simulink library "groundStation001_cl"  (R2018b)
settings: Solver=VariableStepAuto  StartTime=0.0  StopTime=10.0  RelTol=1e-3
values from neighbouring files (symbols this model uses):
  env = ENV.env    [groundStation001_ts.m]    (also in groundStation001_ts2.m; groundStation001_ts3.m)
  gndStn = OCT.sixDoFStation    [groundStation001_ts3.m]
libraries: thrAttachPtKinematics_ul x3, tethersMoment_cl x2, vrlib x1, eulAng2RotMat_ul x1, circulationForce_ul x1, sixDoFDynamics_ul x1, tether000_cl x1, variableBuoyancy_ul x1, winch_cl x1
settings Model: Creator=Erin B  LastModifiedBy=mcobb

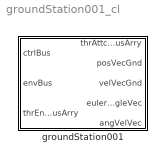
== system groundStation001_cl ==
  groundStation001 : Subsystem  mask{gs=gndStn, e=0, numNodes=0}
      mask prompts: gs "Ground Station"; e "Environmetnt"; numNodes "Number of anchor tether nodes"
      mask init:
      | groundStation001_init

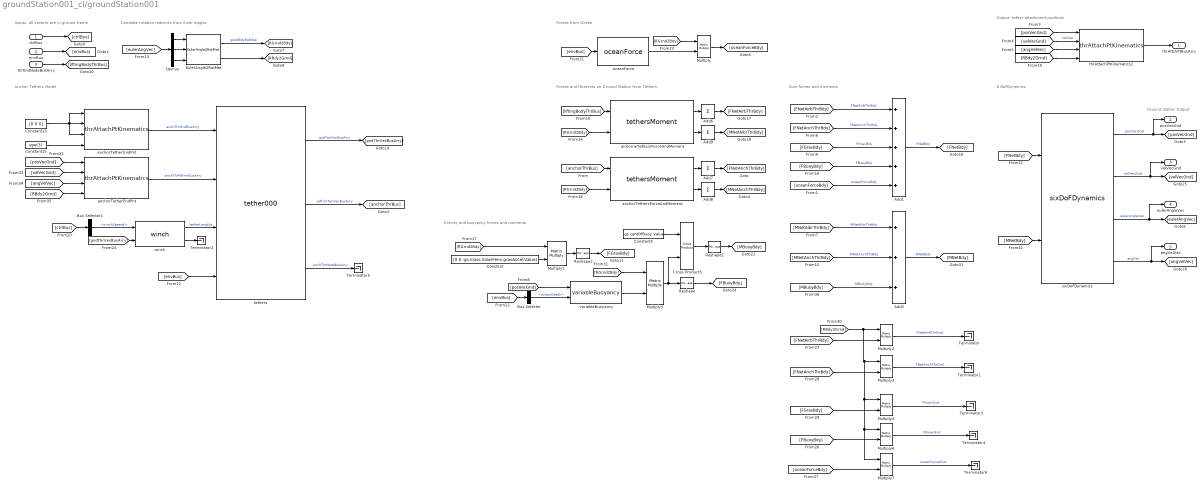
== system groundStation001_cl/groundStation001 ==
  note: Ground Station Output
  note: Anchor Tethers Model
  note: Forces and Moments on Ground Station from Tethers
  note: Output: tether attachment positions
  note: Inputs, all vectors are in ground frame
  note: Calculate rotation matrices from Euler angles
  note: Sum forces and moments
  note: Gravity and buoyancy forces and moments
  note: 6 DoFDynamics
  note: Forces from Ocean
  ctrlBus : Inport  OutDataTypeStr=Bus: gndStnCtrlBus
  envBus : Inport  Port=2  OutDataTypeStr=Bus: envBus
  thrEndNodeBusArry : Inport  Port=3
  Add1 : Sum  Inputs=+++++
  Add2 : Sum  Inputs=+++
  Add{6..9} (4 alike) : Sum  Inputs=+  CollapseMode=Specified dimension  CollapseDim=2
  Bus Selector : BusSelector  OutputSignals=oceanDepth
  Bus Selector1 : BusSelector  OutputSignals=winchSpeeds
  Constant : Constant  Value=[0 0 -gs.mass.Value*env.gravAccel.Value]
  Constant13 : Constant  Value=[0 0 0]
  Constant15 : Constant  Value=eye(3)
  Constant5 : Constant  Value=gs.centOfBuoy.Value
  Cross Product3 : vrlib/Utilities/Cross Product
      settings: SourceProductBaseCode=VR
  Demux : Demux  Outputs=3
  EulerAngle2RotMat : eulAng2RotMat_ul/EulerAngle2RotMat  SystemSampleTime=-1
  Multiply{,1..7} (8 alike) : Product  Multiplication=Matrix(*)
  Reshape : Reshape  OutputDimensionality=Column vector (2-D)
  Reshape1 : Reshape  OutputDimensionality=Column vector (2-D)
  Reshape2 : Reshape  OutputDimensionality=Column vector (2-D)
  Terminator{,1..6} (7 alike) : Terminator
  airborneTethersForceAndMoment : tethersMoment_cl/tethersMoment  arms=gs.struct('OCT.thrAttch','air')
  anchorTetherEndPnt : thrAttachPtKinematics_ul/thrAttachPtKinematics  atchPts=gs.struct('OCT.thrAttch','bdy')
  anchorTetherGndPnt : thrAttachPtKinematics_ul/thrAttachPtKinematics  atchPts=gs.struct('OCT.thrAttch','gnd')
  anchorTethersForceAndMoment : tethersMoment_cl/tethersMoment  arms=gs.struct('OCT.thrAttch','bdy')
  oceanForce : circulationForce_ul/oceanForce  A=gs.volume.Value^(2/3)  cd=gs.dragCoeff.Value
  sixDoFDynamics : sixDoFDynamics_ul/sixDoFDynamics  M=gs.mass.Value  M_added=zeros(3,3)  J=gs.inertiaMatrix.Value  J_added=zeros(3,3)  initPos=gs.initPos.Value  initVel=gs.initVel.Value  initEulAngs=gs.initEulAng.Value  initAngVel=gs.initAngVel.Value
  tethers : tether000_cl/tether000  VariantControl=VSS_tethers_tether000  LabelModeActiveChoice=NNodeTether  numNodes=0  thrStructure=gs.anchThrs.struct('OCT.tether')  fluidDensity=e.water.density.Value  gravity=e.gravAccel.Value
  thrAttachPtKinematics2 : thrAttachPtKinematics_ul/thrAttachPtKinematics  atchPts=gs.struct('OCT.thrAttch','air')
  variableBuoyancy : variableBuoyancy_ul/variableBuoyancy  vol=gs.volume.Value  h=(gs.volume.Value)^(1/3)  rho=e.water.density.Value  grav=e.gravAccel.Value
  winch : winch_cl/winch  SystemSampleTime=-1
  thrAttchPtBusArry : Outport
  posVecGnd : Outport  Port=2
  velVecGnd : Outport  Port=3
  eulerAngleVec : Outport  Port=4
  angVelVec : Outport  Port=5
  wires:
  EulerAngle2RotMat/2 -> [RBdy2Grnd]
  sixDoFDynamics/4 -> angVelVec/1, [angVelVec]  "angVel"
  variableBuoyancy/1 -> Multiply5/2
  [MBuoyBdy] -> Add2/3  "MBuoyBdy"
  [FNetBdy] -> sixDoFDynamics/1
  tethers/3 -> Terminator5/1  "anchThrNodeBusArry"
  anchorTetherGndPnt/1 -> tethers/1  "anchThrGndBusArry"
  Add1/1 -> [FNetBdy]  "FNetBdy"
  Demux/2 -> EulerAngle2RotMat/2
  sixDoFDynamics/2 -> velVecGnd/1, [velVecGnd]  "velVecGnd"
  [envBus] -> tethers/4
  [RGrnd2Bdy] -> Multiply5/1
  tethers/2 -> [anchorThrBus]  "pltfrmTenVecBusArry"
  Cross Product3/1 -> Reshape1/1
  tethers/1 -> [gndThrVecBusArry]  "gndTenVecBusArry"
  sixDoFDynamics/3 -> eulerAngleVec/1, [eulerAngVec]  "eulerAngleVec"
  Multiply1/1 -> Reshape2/1
  Multiply5/1 -> Reshape/1, Cross Product3/2
  Constant/1 -> Multiply1/2
  anchorTetherEndPnt/1 -> tethers/2  "anchThrPltfrmBusArry"
  sixDoFDynamics/1 -> posVecGnd/1, [posVecGnd]  "posVecGnd"
  [RGrnd2Bdy] -> anchorTethersForceAndMoment/2
  Demux/1 -> EulerAngle2RotMat/1
  Constant5/1 -> Cross Product3/1
  [eulerAngVec] -> Demux/1
  Demux/3 -> EulerAngle2RotMat/3
  [RGrnd2Bdy] -> Multiply1/1
  EulerAngle2RotMat/1 -> [RGrnd2Bdy]  "gnd2BdyRotMat"
  [MNetBdy] -> sixDoFDynamics/2
  [posVecGnd] -> variableBuoyancy/1
  [posVecGnd] -> anchorTetherEndPnt/1
  [angVelVec] -> anchorTetherEndPnt/3
  [RBdy2Grnd] -> anchorTetherEndPnt/4
  [velVecGnd] -> anchorTetherEndPnt/2
  Constant13/1 -> anchorTetherGndPnt/3, anchorTetherGndPnt/1, anchorTetherGndPnt/2
  Constant15/1 -> anchorTetherGndPnt/4
  anchorTethersForceAndMoment/1 -> Add7/1
  anchorTethersForceAndMoment/2 -> Add8/1
  Add7/1 -> [FNetAnchThrBdy]
  Add8/1 -> [MNetAnchThrBdy]
  oceanForce/1 -> Multiply/2
  [velVecGnd] -> thrAttachPtKinematics2/2  "velVec"
  [RBdy2Grnd] -> thrAttachPtKinematics2/4
  [angVelVec] -> thrAttachPtKinematics2/3
  [posVecGnd] -> thrAttachPtKinematics2/1
  thrAttachPtKinematics2/1 -> thrAttchPtBusArry/1
  thrEndNodeBusArry/1 -> [liftingBodyThrBus]
  Add2/1 -> [MNetBdy]  "MNetBdy"
  ctrlBus/1 -> [ctrlBus]
  envBus/1 -> [envBus]
  [oceanForceBdy] -> Add1/5  "oceanForceBdy"
  [liftingBodyThrBus] -> airborneTethersForceAndMoment/1
  [RGrnd2Bdy] -> airborneTethersForceAndMoment/2
  Add9/1 -> [MNetAibrThrBdy]
  Add6/1 -> [FNetAirbThrBdy]
  airborneTethersForceAndMoment/1 -> Add6/1
  airborneTethersForceAndMoment/2 -> Add9/1
  [anchorThrBus] -> anchorTethersForceAndMoment/1
  [FGravBdy] -> Add1/3  "FGravBdy"
  [FNetAirbThrBdy] -> Add1/1  "FNetAirbThrBdy"
  [FNetAnchThrBdy] -> Add1/2  "FNetAnchThrBdy"
  [MNetAibrThrBdy] -> Add2/1  "MNetAibrThrBdy"
  [MNetAnchThrBdy] -> Add2/2  "MNetAnchThrBdy"
  [FBuoyBdy] -> Add1/4  "FBuoyBdy"
  winch/1 -> tethers/3  "tetherLengths"
  [gndThrVecBusArry] -> winch/2
  winch/2 -> Terminator2/1
  [ctrlBus] -> Bus Selector1/1
  [envBus] -> oceanForce/1
  [envBus] -> Bus Selector/1
  Bus Selector/1 -> variableBuoyancy/2  "<oceanDepth>"
  Bus Selector1/1 -> winch/1  "<winchSpeeds>"
  Multiply/1 -> [oceanForceBdy]
  [RGrnd2Bdy] -> Multiply/1
  Reshape/1 -> [FBuoyBdy]
  Reshape1/1 -> [MBuoyBdy]
  Reshape2/1 -> [FGravBdy]
  [FNetAirbThrBdy] -> Multiply2/2
  [FNetAnchThrBdy] -> Multiply3/2
  [FGravBdy] -> Multiply4/2
  [FBuoyBdy] -> Multiply6/2
  [oceanForceBdy] -> Multiply7/2
  [RBdy2Grnd] -> Multiply7/1, Multiply6/1, Multiply4/1, Multiply3/1, Multiply2/1
  Multiply2/1 -> Terminator/1  "FNetAirbThrGnd"
  Multiply3/1 -> Terminator1/1  "FNetAnchThrGnd"
  Multiply4/1 -> Terminator3/1  "FGravGnd"
  Multiply6/1 -> Terminator4/1  "FBuoyGnd"
  Multiply7/1 -> Terminator6/1  "oceanForceGnd"
